simulink model "Practica5_2022A"  (R2022a)
settings: Solver=VariableStepAuto  StartTime=0.0  StopTime=10  RelTol=1e-3
settings Model: Creator=edgar  LastModifiedBy=Anahi Monserrat
settings ModelReferenceCC: EnableRefExpFcnMdlSchedulingChecks=off
settings RTWCC: Description=Generic Real-Time Target

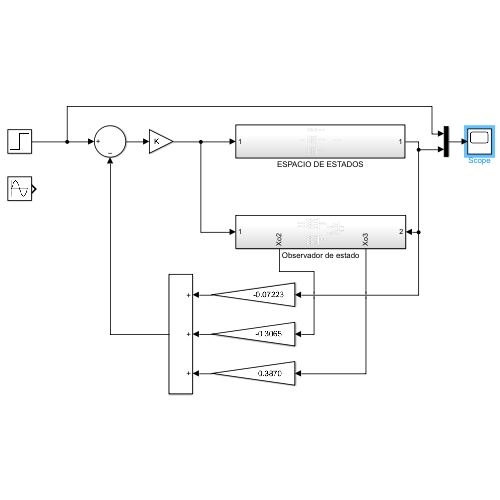
[thumbnail: Simulink's stored preview of the top-level diagram]
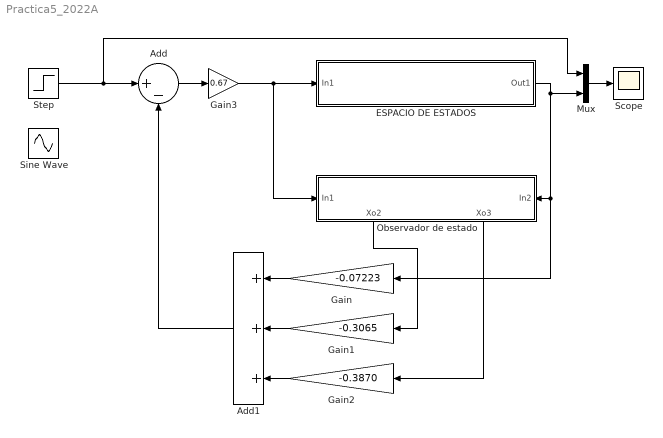
== system Practica5_2022A ==
  Add : Sum  Inputs=|+-
  Add1 : Sum  Inputs=+++
  ESPACIO DE ESTADOS : Subsystem
  Gain : Gain  Gain=-0.07223
  Gain1 : Gain  Gain=-0.3065
  Gain2 : Gain  Gain=-0.3870
  Gain3 : Gain  Gain=0.67
  Mux : Mux  Inputs=2
  Observador de estado : Subsystem
      settings: PortSchema="{\"entries\":[{\"content\":{\"sides\":[{\"content\":{\"connectorIds\":[\"In1\"]},\"type\":\"ConnectorPlacement.EquallySpacedRectSide\",\"uuid\":\"9933af09-e30a-4a3c-a0e3-dffec2223d50\"},{\"content\":{\"connectorIds\":[\"In2\"],\"side\":\"RIGHT\"},\"type\":\"ConnectorPlacement.EquallySpacedRectSide\",\"uuid\":\"a5fb4d5c-b0b2-4fa6-9ed9-ad5917edf078\"},{\"content\":{\"side\":\"TOP\"},\"type\":\"ConnectorPlacement.EquallySpacedRectSide\",\"uuid\":\"6702ee26-218a-4e5a-8b7f-2d20323f3f9e\"},{\"content\":{\"connectorIds\":[\"Out1\",\"Out2\"],\"side\":\"BOTTOM\"},\"type\":\"ConnectorPlacement.EquallySpacedRectSide\",\"uuid\":\"bb15bb68-788c-4e99-a02f-77e7536579be\"}]},\"type\":\"ConnectorPlacement.EquallySpacedConnector\",\"uuid\":\"78becabe-a2b6-43cf-81c2-35f37bc38762\"}],\"packageUris\":[\"http://schema.mathworks.com/mf0/Connector/R2020b\"],\"version\":\"1.0\"}"
  Scope : Scope
  Sine Wave : Sin  SampleTime=0
  Step : Step  SampleTime=0
  wires:
  Add1/1 -> Add/2
  Mux/1 -> Scope/1
  Add/1 -> Gain3/1
  Gain1/1 -> Add1/2
  Step/1 -> Add/1, Mux/1
  ESPACIO DE ESTADOS/1(Out1) -> Mux/2, Gain/1, Observador de estado/2(In2)
  Gain/1 -> Add1/1
  Gain2/1 -> Add1/3
  Observador de estado/1(Xo2) -> Gain1/1
  Observador de estado/2(Xo3) -> Gain2/1
  Gain3/1 -> ESPACIO DE ESTADOS/1(In1), Observador de estado/1(In1)

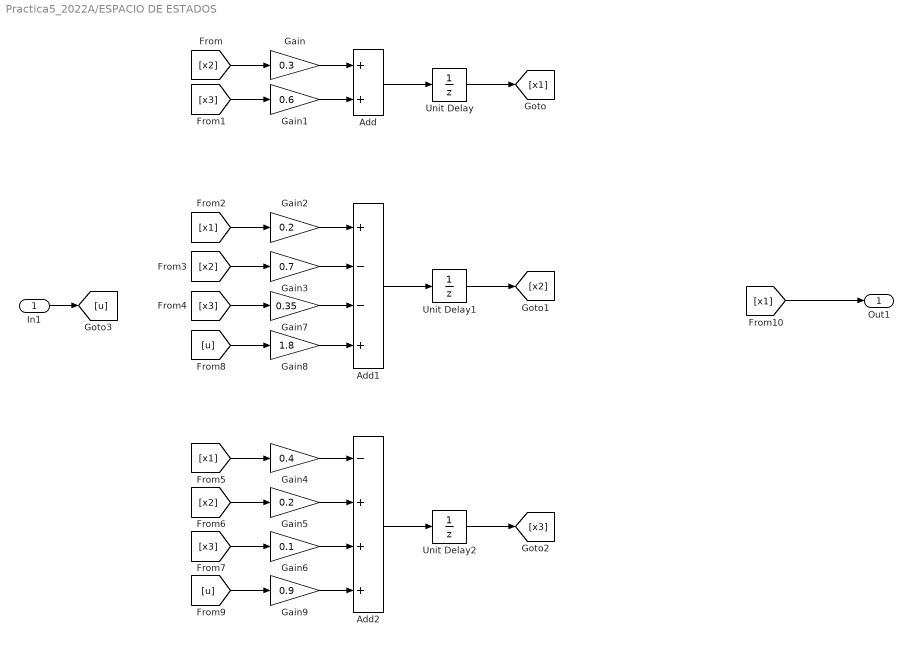
== system Practica5_2022A/ESPACIO DE ESTADOS ==
  In1 : Inport
  Add : Sum
  Add1 : Sum  Inputs=+--+
  Add2 : Sum  Inputs=-+++
  Gain : Gain  Gain=0.3
  Gain1 : Gain  Gain=0.6
  Gain2 : Gain  Gain=0.2
  Gain3 : Gain  Gain=0.7
  Gain4 : Gain  Gain=0.4
  Gain5 : Gain  Gain=0.2
  Gain6 : Gain  Gain=0.1
  Gain7 : Gain  Gain=0.35
  Gain8 : Gain  Gain=1.8
  Gain9 : Gain  Gain=0.9
  Unit Delay : UnitDelay  SampleTime=-1  HasFrameUpgradeWarning=on
  Unit Delay1 : UnitDelay  SampleTime=-1  HasFrameUpgradeWarning=on
  Unit Delay2 : UnitDelay  SampleTime=-1  HasFrameUpgradeWarning=on
  Out1 : Outport
  wires:
  Unit Delay/1 -> [x1]
  Unit Delay1/1 -> [x2]
  Unit Delay2/1 -> [x3]
  Add2/1 -> Unit Delay2/1
  Add1/1 -> Unit Delay1/1
  Add/1 -> Unit Delay/1
  Gain/1 -> Add/1
  Gain1/1 -> Add/2
  Gain7/1 -> Add1/3
  Gain3/1 -> Add1/2
  Gain2/1 -> Add1/1
  Gain5/1 -> Add2/2
  Gain4/1 -> Add2/1
  Gain6/1 -> Add2/3
  [x2] -> Gain/1
  [x3] -> Gain1/1
  [x1] -> Gain2/1
  [x2] -> Gain3/1
  [x3] -> Gain7/1
  [x1] -> Gain4/1
  [x2] -> Gain5/1
  [x3] -> Gain6/1
  In1/1 -> [u]
  Gain9/1 -> Add2/4
  [u] -> Gain9/1
  [u] -> Gain8/1
  Gain8/1 -> Add1/4
  [x1] -> Out1/1

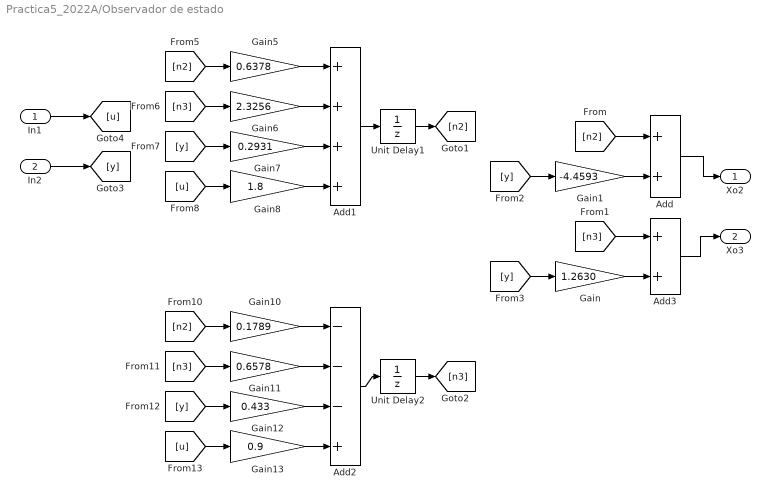
== system Practica5_2022A/Observador de estado ==
  In1 : Inport
  In2 : Inport  Port=2
  Add : Sum
  Add1 : Sum  Inputs=++++
  Add2 : Sum  Inputs=---+
  Add3 : Sum
  Gain : Gain  Gain=1.2630
  Gain1 : Gain  Gain=-4.4593
  Gain10 : Gain  Gain=0.1789
  Gain11 : Gain  Gain=0.6578
  Gain12 : Gain  Gain=0.433
  Gain13 : Gain  Gain=0.9
  Gain5 : Gain  Gain=0.6378
  Gain6 : Gain  Gain=2.3256
  Gain7 : Gain  Gain=0.2931
  Gain8 : Gain  Gain=1.8
  Unit Delay1 : UnitDelay  SampleTime=-1  HasFrameUpgradeWarning=on
  Unit Delay2 : UnitDelay  SampleTime=-1  HasFrameUpgradeWarning=on
  Xo2 : Outport
  Xo3 : Outport  Port=2
  wires:
  Unit Delay1/1 -> [n2]
  Unit Delay2/1 -> [n3]
  In2/1 -> [y]
  In1/1 -> [u]
  [n2] -> Gain5/1
  [y] -> Gain7/1
  [n3] -> Gain6/1
  Add1/1 -> Unit Delay1/1
  [u] -> Gain8/1
  [u] -> Gain13/1
  [n3] -> Gain11/1
  [y] -> Gain12/1
  [n2] -> Gain10/1
  Add2/1 -> Unit Delay2/1
  Gain8/1 -> Add1/4
  Gain7/1 -> Add1/3
  Gain6/1 -> Add1/2
  Gain5/1 -> Add1/1
  Gain13/1 -> Add2/4
  Gain12/1 -> Add2/3
  Gain11/1 -> Add2/2
  Gain10/1 -> Add2/1
  Add/1 -> Xo2/1
  Add3/1 -> Xo3/1
  [n2] -> Add/1
  [n3] -> Add3/1
  Gain/1 -> Add3/2
  Gain1/1 -> Add/2
  [y] -> Gain1/1
  [y] -> Gain/1
